simulink model "train_model"  (Simulink 8.9)
settings: Solver=FixedStepDiscrete  StartTime=0.0  StopTime=10.0  FixedStep=1  MaxStep=1  RelTol=1e-3
model workspace (MAT data in the model file):
  CLSRN = Simulink.Signal
  CLSRN.DataType = 'auto'
  CLSRN.Dimensions = -1
  CLSRN.DimensionsMode = 'auto'
  CLSRN.Complexity = 'auto'
  CLSRN.SampleTime = -1
  CLSRN.SamplingMode = 'auto'
libraries: simulink x8
settings Model: Creator=Natasha  LastModifiedBy=Natasha
settings DataIOCC: LimitDataPoints=off  SaveFormat=Dataset  SignalLoggingSaveFormat=Dataset  ReturnWorkspaceOutputs=on
settings OptimizationCC: DefaultParameterBehavior=Inlined  UseDivisionForNetSlopeComputation=on  UseFloatMulNetSlope=on  InlineInvariantSignals=on  PassReuseOutputArgsAs=Individual arguments  ZeroExternalMemoryAtStartup=off  ZeroInternalMemoryAtStartup=off  NoFixptDivByZeroProtection=on  EfficientFloat2IntCast=on  LifeSpan=1  OptimizeBlockOrder=speed
settings DebuggingCC: UnderspecifiedInitializationDetection=Simplified  MergeDetectMultiDrivingBlocksExec=error  ParameterTunabilityLossMsg=error  FcnCallInpInsideContextMsg=error  StateNameClashWarn=none  SFUnexpectedBacktrackingDiag=error  SFNoUnconditionalDefaultTransitionDiag=error  SFExecutionAtInitializationDiag=warning
settings HardwareCC: ProdBitPerPointer=64  ProdBitPerSizeT=64  ProdBitPerPtrDiffT=64  ProdLargestAtomicFloat=Float  ProdIntDivRoundTo=Zero  ProdEndianess=LittleEndian  ProdWordSize=64  ProdLongLongMode=on  ProdHWDeviceType=Intel->x86-64 (Windows64)
settings ModelReferenceCC: PropagateSignalLabelsOutOfModel=on
settings SFSimCC: SimUseLocalCustomCode=on  MATLABDynamicMemAlloc=off
settings RTWCC: SystemTargetFile=ert.tlc  TemplateMakefile=ert_default_tmf  Description=Embedded Coder  GenerateReport=on  RTWUseLocalCustomCode=on  IncludeHyperlinkInReport=on  LaunchReport=on  GenerateTraceInfo=on  GenerateTraceReport=on  GenerateTraceReportSl=on  GenerateTraceReportSf=on  GenerateTraceReportEml=on  GenerateCodeMetricsReport=on
settings CodeAppCC: ForceParamTrailComments=on  IgnoreCustomStorageClasses=off  OperatorAnnotations=on  SimulinkDataObjDesc=on  SFDataObjDesc=on  CustomSymbolStrGlobalVar=rt$N$M  CustomSymbolStrType=$N$M  CustomSymbolStrFcn=$N$M$F  CustomSymbolStrMacro=$N$M  InsertBlockDesc=on
settings ERTTargetCC: TargetLangStandard=C99 (ISO)  GenerateSampleERTMain=on  IncludeMdlTerminateFcn=off  CombineSignalStateStructs=on  SupportAbsoluteTime=off  SupportComplex=off  SupportNonInlinedSFcns=on  InlinedParameterPlacement=NonHierarchical  ERTCustomFileTemplate=example_file_process.tlc  ERTFilePackagingFormat=CompactWithDataFile
settings ConfigComp: CovMetricSettings=dwe  CovHtmlReporting=off  CovSaveCumulativeToWorkspaceVar=off  CovSaveSingleToWorkspaceVar=off  CovExternalEMLEnable=on

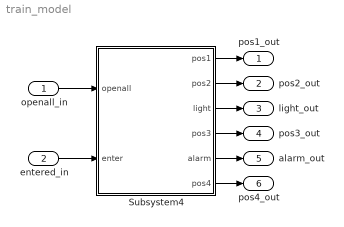
== system train_model ==
  "openall_in " : Inport
  "entered_in " : Inport  Port=2
  Subsystem4 : Subsystem
  "pos1_out " : Outport
  "pos2_out " : Outport  Port=2
  "light_out " : Outport  Port=3
  "pos3_out " : Outport  Port=4
  "alarm_out " : Outport  Port=5
  pos4_out : Outport  Port=6
  wires:
  "openall_in "/1 -> Subsystem4/1("openall ")
  "entered_in "/1 -> Subsystem4/2("enter ")
  Subsystem4/1(pos1) -> "pos1_out "/1
  Subsystem4/2("pos2 ") -> "pos2_out "/1
  Subsystem4/3(light) -> "light_out "/1
  Subsystem4/4("pos3 ") -> "pos3_out "/1
  Subsystem4/5(alarm) -> "alarm_out "/1
  Subsystem4/6("pos4 ") -> pos4_out/1

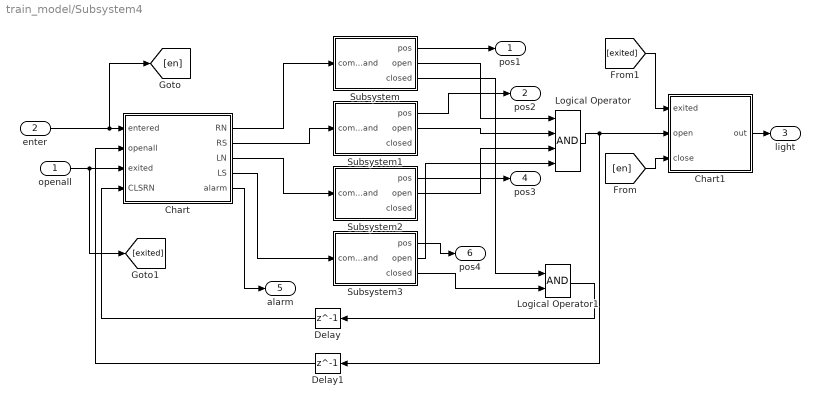
== system train_model/Subsystem4 ==
  "openall " : Inport
  "enter " : Inport  Port=2
  Chart : Stateflow chart  TreatAsAtomicUnit=on
  Chart1 : Stateflow chart  TreatAsAtomicUnit=on
  Delay : Delay  DelayLength=1  InitialCondition=0  UseCircularBuffer=on
  Delay1 : Delay  DelayLength=1  InitialCondition=0  UseCircularBuffer=on
  Logical Operator : Logic  Inputs=4  AllPortsSameDT=off  OutDataTypeStr=boolean
  Logical Operator1 : Logic  AllPortsSameDT=off  OutDataTypeStr=boolean
  Subsystem : Subsystem
  Subsystem1 : Subsystem
  Subsystem2 : Subsystem
  Subsystem3 : Subsystem
  pos1 : Outport
  "pos2 " : Outport  Port=2
  light : Outport  Port=3
  "pos3 " : Outport  Port=4
  alarm : Outport  Port=5
  "pos4 " : Outport  Port=6
  wires:
  Subsystem/2(open) -> Logical Operator/1
  Logical Operator/1 -> Delay1/1, Chart1/2(open)
  Subsystem2/2(open) -> Logical Operator/3
  "enter "/1 -> [en], Chart/1(entered)
  "openall "/1 -> [exited], Chart/3(exited)
  Subsystem1/2(open) -> Logical Operator/2
  Subsystem1/1("pos ") -> "pos2 "/1
  Chart/2(RS) -> Subsystem1/1(command)
  [exited] -> Chart1/1(exited)
  Delay/1 -> Chart/4(CLSRN)
  Chart/1(RN) -> Subsystem/1(command)
  Chart/4(LS) -> Subsystem3/1(command)
  Subsystem3/2(open) -> Logical Operator/4
  Chart/3(LN) -> Subsystem2/1(command)
  [en] -> Chart1/3(close)
  Subsystem/1("pos ") -> pos1/1
  Subsystem2/1("pos ") -> "pos3 "/1
  Subsystem3/3(closed) -> Logical Operator1/2
  Subsystem3/1("pos ") -> "pos4 "/1
  Chart1/1(out) -> light/1
  Subsystem/3(closed) -> Logical Operator1/1
  Chart/5(alarm) -> alarm/1
  Logical Operator1/1 -> Delay/1
  Delay1/1 -> Chart/2(openall)

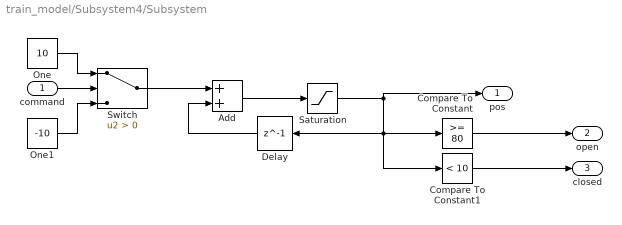
== system train_model/Subsystem4/Subsystem ==
  command : Inport  OutDataTypeStr=boolean
  Add : Sum
  Compare To Constant : simulink/Logic and Bit Operations/Compare To Constant  relop=>=  const=80  OutDataTypeStr=boolean
  Compare To Constant1 : simulink/Logic and Bit Operations/Compare To Constant  relop=<  const=10  OutDataTypeStr=boolean
  Delay : Delay  DelayLength=1  InitialCondition=0
  One : Constant  Value=10  OutDataTypeStr=Inherit: Inherit via back propagation
  One1 : Constant  Value=-10  OutDataTypeStr=Inherit: Inherit via back propagation
  Saturation : Saturate  UpperLimit=90  LowerLimit=0
  Switch : Switch  Criteria=u2 > Threshold
  "pos " : Outport
  open : Outport  Port=2
  closed : Outport  Port=3
  wires:
  Delay/1 -> Add/2
  One/1 -> Switch/1
  Compare To Constant1/1 -> closed/1
  Switch/1 -> Add/1
  Compare To Constant/1 -> open/1
  Saturation/1 -> "pos "/1, Compare To Constant1/1, Compare To Constant/1, Delay/1
  command/1 -> Switch/2
  Add/1 -> Saturation/1
  One1/1 -> Switch/3

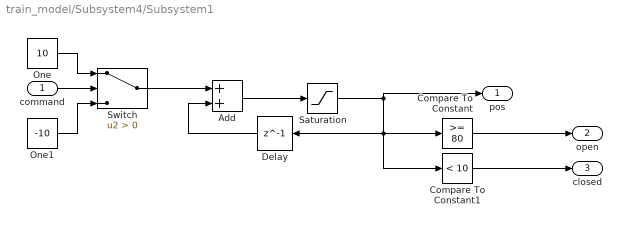
== system train_model/Subsystem4/Subsystem1 ==
  command : Inport
  Add : Sum
  Compare To Constant : simulink/Logic and Bit Operations/Compare To Constant  relop=>=  const=80  OutDataTypeStr=boolean
  Compare To Constant1 : simulink/Logic and Bit Operations/Compare To Constant  relop=<  const=10  OutDataTypeStr=boolean
  Delay : Delay  DelayLength=1  InitialCondition=0
  One : Constant  Value=10  OutDataTypeStr=Inherit: Inherit via back propagation
  One1 : Constant  Value=-10  OutDataTypeStr=Inherit: Inherit via back propagation
  Saturation : Saturate  UpperLimit=90  LowerLimit=0
  Switch : Switch  Criteria=u2 > Threshold
  "pos " : Outport
  open : Outport  Port=2
  closed : Outport  Port=3
  wires:
  One1/1 -> Switch/3
  Add/1 -> Saturation/1
  command/1 -> Switch/2
  Saturation/1 -> Delay/1, Compare To Constant/1, Compare To Constant1/1, "pos "/1
  Compare To Constant/1 -> open/1
  Switch/1 -> Add/1
  Compare To Constant1/1 -> closed/1
  One/1 -> Switch/1
  Delay/1 -> Add/2

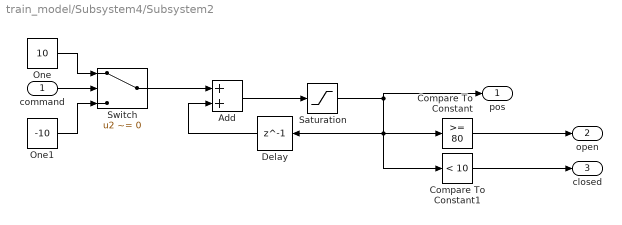
== system train_model/Subsystem4/Subsystem2 ==
  command : Inport
  Add : Sum
  Compare To Constant : simulink/Logic and Bit Operations/Compare To Constant  relop=>=  const=80  OutDataTypeStr=boolean
  Compare To Constant1 : simulink/Logic and Bit Operations/Compare To Constant  relop=<  const=10  OutDataTypeStr=boolean
  Delay : Delay  DelayLength=1  InitialCondition=0
  One : Constant  Value=10  OutDataTypeStr=Inherit: Inherit via back propagation
  One1 : Constant  Value=-10  OutDataTypeStr=Inherit: Inherit via back propagation
  Saturation : Saturate  UpperLimit=90  LowerLimit=0
  Switch : Switch  Criteria=u2 ~= 0
  "pos " : Outport
  open : Outport  Port=2
  closed : Outport  Port=3
  wires:
  Delay/1 -> Add/2
  One/1 -> Switch/1
  Compare To Constant1/1 -> closed/1
  Switch/1 -> Add/1
  Compare To Constant/1 -> open/1
  Saturation/1 -> "pos "/1, Compare To Constant1/1, Compare To Constant/1, Delay/1
  command/1 -> Switch/2
  Add/1 -> Saturation/1
  One1/1 -> Switch/3

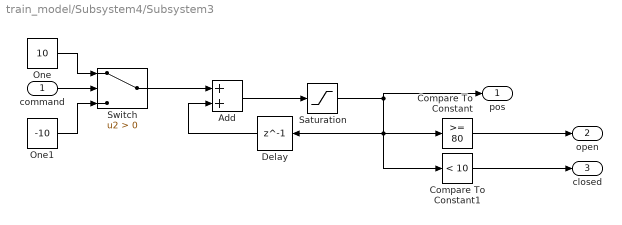
== system train_model/Subsystem4/Subsystem3 ==
  command : Inport
  Add : Sum
  Compare To Constant : simulink/Logic and Bit Operations/Compare To Constant  relop=>=  const=80  OutDataTypeStr=boolean
  Compare To Constant1 : simulink/Logic and Bit Operations/Compare To Constant  relop=<  const=10  OutDataTypeStr=boolean
  Delay : Delay  DelayLength=1  InitialCondition=0
  One : Constant  Value=10  OutDataTypeStr=Inherit: Inherit via back propagation
  One1 : Constant  Value=-10  OutDataTypeStr=Inherit: Inherit via back propagation
  Saturation : Saturate  UpperLimit=90  LowerLimit=0
  Switch : Switch  Criteria=u2 > Threshold
  "pos " : Outport
  open : Outport  Port=2
  closed : Outport  Port=3
  wires:
  One1/1 -> Switch/3
  Add/1 -> Saturation/1
  command/1 -> Switch/2
  Saturation/1 -> Delay/1, Compare To Constant/1, Compare To Constant1/1, "pos "/1
  Compare To Constant/1 -> open/1
  Switch/1 -> Add/1
  Compare To Constant1/1 -> closed/1
  One/1 -> Switch/1
  Delay/1 -> Add/2

== stateflow chart Subsystem4/Chart1 ==
  state orange_open
    en:
    out = 2;
  state Green
    en:
    out = 1;
  state orange_close
    en:
    out = 2;
    count = 0;
    du:
    count = count + 1;
  state Red
    en:
    out = 3;
  (default) -> Green
  orange_open -> Green : [open]
  Red -> orange_open : [exited]
  Green -> orange_close : [close]
  orange_close -> Red : [count >= 4]
  data: exited input double; open input double; out output double; count local double; close input double

== stateflow chart Subsystem4/Chart ==
  state Openall
    en:
    LN = false;
    LS = false;
    RN = false;
    RS = false;
    STATEPOS = 5;
    count = 0;
    du:
    count = count + 1
  state Opened
    en:
    LN = true;
    LS = true;
    RN = true;
    RS = true;
    STATEPOS = 1;
    alarm = false;
  state alert
    en, du: alarm = true;
  state LNRS
    en:
    LN = false;
    RS = false;
    count = 0;
    STATEPOS = 4;
    du:
    count = count+1
  state entered
    en:
    LS = false;
    RN = false;
    STATEPOS = 2;
    count = 0;
    du:
    count = count + 1;
  state closedLSRN
    en:
    count = 0;
    STATEPOS = 3;
    du:
    count = count +1
  Openall -> Opened [order 1] : [openall]
  (default) -> Opened
  Openall -> alert [order 2] : [count > 12]
  LNRS -> Openall : [exited]
  alert -> Openall [order 2] : [STATEPOS == 4 && exited]
  Opened -> entered : [entered]
  entered -> alert [order 1] : [count > 12]
  alert -> closedLSRN [order 1] : [STATEPOS == 2 && CLSRN]
  closedLSRN -> LNRS : [count>4]
  entered -> closedLSRN [order 2] : [CLSRN]
  data: entered input boolean; openall input boolean; exited input boolean; RN output boolean; RS output boolean; LN output boolean; LS output boolean; alarm output boolean; STATEPOS local uint32; count local uint32; CLSRN input boolean
